simulink model "NeuromuscularModelwImpedance"  (R2014b)
settings: Solver=ode15s  StartTime=0.0  StopTime=20  MaxStep=.01  RelTol=1e-4  AbsTol=1e-6
values from neighbouring files (symbols this model uses):
  ankleAngleThr = 2*pi/180    (= 0.0349065850399)    [ControlParams.m]    (also in assignGains.m = Gains(48); saveInitialGuess.m = Gains(40))
  bKneeSwing1 = 0.02    [ControlParams.m]    (also in assignGains.m = Gains(36); saveInitialGuess.m = Gains(28))
  bKneeSwing2 = 0.03    [ControlParams.m]    (also in assignGains.m = Gains(37); saveInitialGuess.m = Gains(29))
  k1AnkleStance1 = 5*180/pi    (= 286.478897565)    [ControlParams.m]    (also in assignGains.m = Gains(38); saveInitialGuess.m = Gains(30))
  k1AnkleStance2 = 5*180/pi    (= 286.478897565)    [ControlParams.m]    (also in assignGains.m = Gains(39); saveInitialGuess.m = Gains(31))
  k1AnkleSwing1 = .5*180/pi    (= 28.6478897565)    [ControlParams.m]    (also in assignGains.m = Gains(40); saveInitialGuess.m = Gains(32))
  k1AnkleSwing2 = 0.75*180/pi    (= 42.9718346348)    [ControlParams.m]    (also in assignGains.m = Gains(41); saveInitialGuess.m = Gains(33))
  k1KneeStance1 = 3.7*180/pi    (= 211.994384198)    [ControlParams.m]    (also in assignGains.m = Gains(42); saveInitialGuess.m = Gains(34))
  k1KneeStance2 = 2.53*180/pi    (= 144.958322168)    [ControlParams.m]    (also in assignGains.m = Gains(43); saveInitialGuess.m = Gains(35))
  k1KneeSwing1 = 0.05*180/pi    (= 2.86478897565)    [ControlParams.m]    (also in assignGains.m = Gains(44); saveInitialGuess.m = Gains(36))
  k1KneeSwing2 = 2.3*180/pi    (= 131.78029288)    [ControlParams.m]    (also in assignGains.m = Gains(45); saveInitialGuess.m = Gains(37))
  k2AnkleStance1 = .5*(180/pi)^3    (= 94045.4744072)    [ControlParams.m]    (also in assignGains.m = Gains(46); saveInitialGuess.m = Gains(38))
  k2KneeStance2 = 7e-4*(180/pi)^3    (= 131.66366417)    [ControlParams.m]    (also in assignGains.m = Gains(47); saveInitialGuess.m = Gains(39))
  LceOffsetTA = 1-0.5*w    [ControlParams.m]
  legLengthClr = .9    (= 0.9)    [ControlParams.m]    (also in assignGains.m = Gains(56); saveInitialGuess.m = Gains(48))
  LongDelay = 0.020    (= 0.02)    [ControlParams.m]
  MidDelay = 0.010    (= 0.01)    [ControlParams.m]
  phiAnkleStance1 = 5*pi/180    (= 0.0872664625997)    [ControlParams.m]    (also in assignGains.m = Gains(49); saveInitialGuess.m = Gains(41))
  phiAnkleStance12 = 2*pi/180    (= 0.0349065850399)    [ControlParams.m]    (also in assignGains.m = Gains(50); saveInitialGuess.m = Gains(42))
  phiAnkleStance2 = 10*pi/180    (= 0.174532925199)    [ControlParams.m]    (also in assignGains.m = Gains(51); saveInitialGuess.m = Gains(43))
  phiHATref = 6*pi/180    (= 0.10471975512)    [ControlParams.m]
  phiKneeStance1 = 8*pi/180    (= 0.13962634016)    [ControlParams.m]    (also in assignGains.m = Gains(52); saveInitialGuess.m = Gains(44))
  phiKneeStance2 = 16*pi/180    (= 0.279252680319)    [ControlParams.m]    (also in assignGains.m = Gains(53); saveInitialGuess.m = Gains(45))
  phiKneeSwing1 = 65*pi/180    (= 1.1344640138)    [ControlParams.m]    (also in assignGains.m = Gains(54); saveInitialGuess.m = Gains(46))
  phiKneeSwing2 = 40*pi/180    (= 0.698131700798)    [ControlParams.m]    (also in assignGains.m = Gains(55); saveInitialGuess.m = Gains(47))
  PreStimGG = 0.05    [ControlParams.m]
  PreStimGLU = 0.01    [ControlParams.m]
  PreStimHAM = 0.01    [ControlParams.m]
  ShortDelay = 0.005    [ControlParams.m]
  simbiconGainD = 5*pi/180    (= 0.0872664625997)    [ControlParams.m]    (also in assignGains.m = Gains(57); saveInitialGuess.m = Gains(49))
  simbiconGainV = 5*pi/180    (= 0.0872664625997)    [ControlParams.m]    (also in assignGains.m = Gains(58); saveInitialGuess.m = Gains(50))
  simbiconLegAngle0 = 85*pi/180    (= 1.4835298642)    [ControlParams.m]    (also in assignGains.m = Gains(59); saveInitialGuess.m = Gains(51))
undefined symbols (not defined in the file or in its folder): DeltaThRef, footCenterToCGDist, footInertia, footMass, g, loptGAS, loptHAMCut, loptTA, lslackGAS, lslackHAMCut, phimaxGASa, phimaxGASk, phirefGASa, phirefGASk, phirefHAMh, rGASa, rGASk, rHAMh, rhoGASa, rhoGASk, rhoHAMh, X, Y, Z
undefined symbols (not defined in the file): RGainGLU, RGainHAM, RhipDGain, RhipPGain, RKglu, RlegAngleFilter, RPosGainGG, RSpeedGainGG
libraries: NeuroMuscularLibrary x67, nesl_utility x16, sm_lib x14, simulink x5, dspswit3 x5, simulink_extras x2
(part 2 of 2)

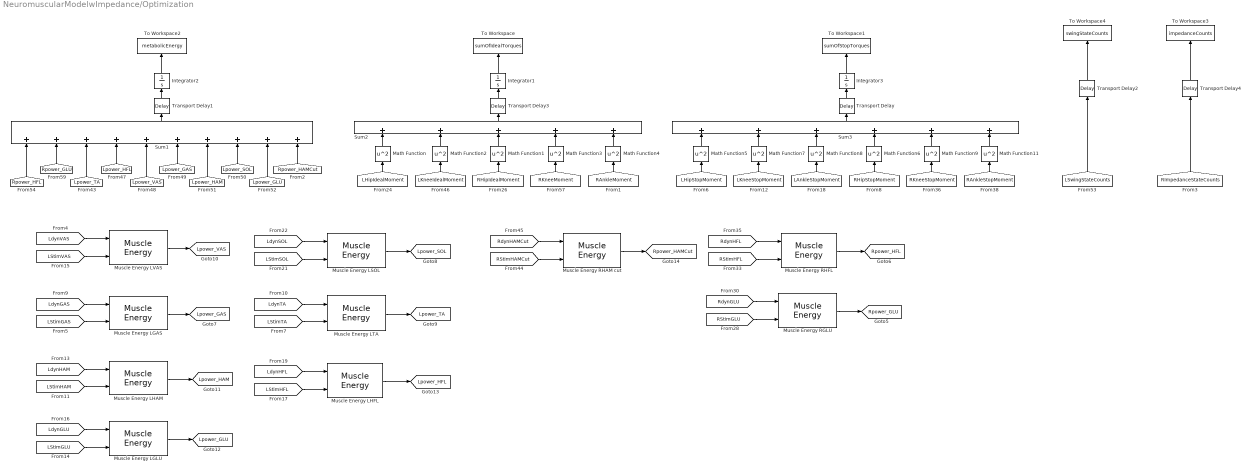
== system NeuromuscularModelwImpedance/Optimization ==
  Integrator1 : Integrator
  Integrator2 : Integrator
  Integrator3 : Integrator
  Math Function{,1..9,11} (11 alike) : Math  Operator=square  SaturateOnIntegerOverflow=on
  Muscle Energy LGAS : NeuroMuscularLibrary/Muscle Energy  lopt=loptGAS  FT=FT_GAS  Fmax=FmaxGAS
  Muscle Energy LGLU : NeuroMuscularLibrary/Muscle Energy  lopt=loptGLU  FT=FT_GLU  Fmax=FmaxGLU
  Muscle Energy LHAM : NeuroMuscularLibrary/Muscle Energy  lopt=loptHAM  FT=FT_HAM  Fmax=FmaxHAM
  Muscle Energy LHFL : NeuroMuscularLibrary/Muscle Energy  lopt=loptHFL  FT=FT_HFL  Fmax=FmaxHFL
  Muscle Energy LSOL : NeuroMuscularLibrary/Muscle Energy  lopt=loptSOL  FT=FT_SOL  Fmax=FmaxSOL
  Muscle Energy LTA : NeuroMuscularLibrary/Muscle Energy  lopt=loptTA  FT=FT_TA  Fmax=FmaxTA
  Muscle Energy LVAS : NeuroMuscularLibrary/Muscle Energy  lopt=loptVAS  FT=FT_VAS  Fmax=FmaxVAS
  Muscle Energy RGLU : NeuroMuscularLibrary/Muscle Energy  lopt=loptGLU  FT=FT_GLU  Fmax=FmaxGLU
  Muscle Energy RHAM cut : NeuroMuscularLibrary/Muscle Energy  lopt=loptHAMCut  FT=FT_HAM  Fmax=FmaxHAMCut
  Muscle Energy RHFL : NeuroMuscularLibrary/Muscle Energy  lopt=loptHFL  FT=FT_HFL  Fmax=FmaxHFL
  Sum1 : Sum  Inputs=++++++++++
  Sum2 : Sum  Inputs=+++++
  Sum3 : Sum  Inputs=++++++
  To Workspace : ToWorkspace  VariableName=sumOfIdealTorques  SampleTime=-1
      settings: MaxDataPoints=1
  To Workspace1 : ToWorkspace  VariableName=sumOfStopTorques  SampleTime=-1
      settings: MaxDataPoints=1
  To Workspace2 : ToWorkspace  VariableName=metabolicEnergy  SampleTime=-1
      settings: MaxDataPoints=1
  To Workspace3 : ToWorkspace  VariableName=impedanceCounts  SampleTime=-1
      settings: MaxDataPoints=1
  To Workspace4 : ToWorkspace  VariableName=swingStateCounts  SampleTime=-1
      settings: MaxDataPoints=1
  Transport Delay : TransportDelay  DelayTime=3  BufferSize=57344
  Transport Delay1 : TransportDelay  DelayTime=3  BufferSize=57344
  Transport Delay2 : TransportDelay  DelayTime=3  BufferSize=24576
  Transport Delay3 : TransportDelay  DelayTime=3  BufferSize=24576
  Transport Delay4 : TransportDelay  DelayTime=3  BufferSize=24576
  tag scope: Lpower_GAS=global, Lpower_GLU=global, Lpower_HAM=global, Lpower_HFL=global, Lpower_SOL=global, Lpower_TA=global, Lpower_VAS=global, Rpower_GLU=global, Rpower_HAMCut=global, Rpower_HFL=global
  wires:
  [RdynGLU] -> Muscle Energy RGLU/1
  [RStimGLU] -> Muscle Energy RGLU/2
  [RdynHFL] -> Muscle Energy RHFL/1
  [RStimHFL] -> Muscle Energy RHFL/2
  Muscle Energy RGLU/1 -> [Rpower_GLU]
  Muscle Energy RHFL/1 -> [Rpower_HFL]
  [LdynSOL] -> Muscle Energy LSOL/1
  [LStimSOL] -> Muscle Energy LSOL/2
  [LStimVAS] -> Muscle Energy LVAS/2
  [LStimGAS] -> Muscle Energy LGAS/2
  Muscle Energy LVAS/1 -> [Lpower_VAS]
  Muscle Energy LGAS/1 -> [Lpower_GAS]
  Muscle Energy LSOL/1 -> [Lpower_SOL]
  Muscle Energy LTA/1 -> [Lpower_TA]
  [LdynTA] -> Muscle Energy LTA/1
  [LStimTA] -> Muscle Energy LTA/2
  [LdynHAM] -> Muscle Energy LHAM/1
  [LStimHAM] -> Muscle Energy LHAM/2
  [LdynGLU] -> Muscle Energy LGLU/1
  [LStimGLU] -> Muscle Energy LGLU/2
  [LdynHFL] -> Muscle Energy LHFL/1
  [LStimHFL] -> Muscle Energy LHFL/2
  Muscle Energy LHAM/1 -> [Lpower_HAM]
  Muscle Energy LGLU/1 -> [Lpower_GLU]
  Muscle Energy LHFL/1 -> [Lpower_HFL]
  [LdynGAS] -> Muscle Energy LGAS/1
  [LdynVAS] -> Muscle Energy LVAS/1
  [RdynHAMCut] -> Muscle Energy RHAM cut/1
  [RStimHAMCut] -> Muscle Energy RHAM cut/2
  Muscle Energy RHAM cut/1 -> [Rpower_HAMCut]
  Integrator2/1 -> To Workspace2/1
  [Rpower_HFL] -> Sum1/1
  [Rpower_GLU] -> Sum1/2
  [Lpower_TA] -> Sum1/3
  [Lpower_HFL] -> Sum1/4
  [Lpower_VAS] -> Sum1/5
  [Lpower_GAS] -> Sum1/6
  [Lpower_HAM] -> Sum1/7
  [Lpower_SOL] -> Sum1/8
  [Lpower_GLU] -> Sum1/9
  Integrator1/1 -> To Workspace/1
  Math Function/1 -> Sum2/1
  [LHipIdealMoment] -> Math Function/1
  Math Function2/1 -> Sum2/2
  [LKneeIdealMoment] -> Math Function2/1
  [RHipIdealMoment] -> Math Function1/1
  Math Function1/1 -> Sum2/3
  [RKneeMoment] -> Math Function3/1
  Math Function3/1 -> Sum2/4
  [RAnkleMoment] -> Math Function4/1
  Math Function4/1 -> Sum2/5
  [Rpower_HAMCut] -> Sum1/10
  Integrator3/1 -> To Workspace1/1
  Math Function5/1 -> Sum3/1
  [LHipStopMoment] -> Math Function5/1
  Math Function7/1 -> Sum3/2
  [LKneeStopMoment] -> Math Function7/1
  [RHipStopMoment] -> Math Function6/1
  Math Function8/1 -> Sum3/3
  [LAnkleStopMoment] -> Math Function8/1
  Math Function6/1 -> Sum3/4
  Sum3/1 -> Transport Delay/1
  Transport Delay/1 -> Integrator3/1
  Sum1/1 -> Transport Delay1/1
  Transport Delay1/1 -> Integrator2/1
  Transport Delay3/1 -> Integrator1/1
  Sum2/1 -> Transport Delay3/1
  [LSwingStateCounts] -> Transport Delay2/1
  Transport Delay2/1 -> To Workspace4/1
  [RImpedanceStateCounts] -> Transport Delay4/1
  Transport Delay4/1 -> To Workspace3/1
  [RKneeStopMoment] -> Math Function9/1
  Math Function9/1 -> Sum3/5
  [RAnkleStopMoment] -> Math Function11/1
  Math Function11/1 -> Sum3/6

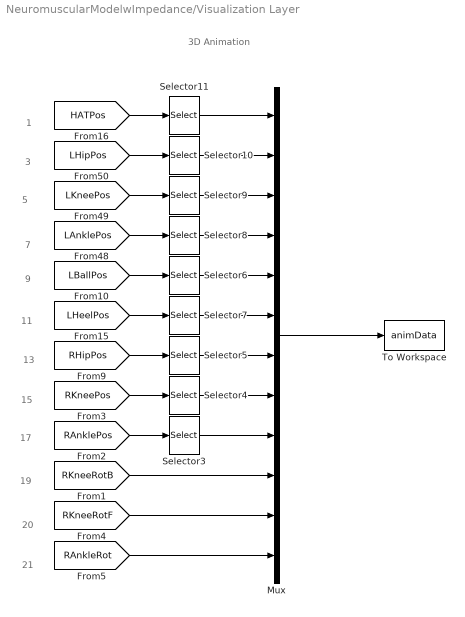
== system NeuromuscularModelwImpedance/Visualization Layer ==
  note: 20
  note: 19
  note: 17
  note: 15
  note: 13
  note: 11
  note: 9
  note: 7
  note: 5
  note: 3
  note: 1
  note: 3D Animation
  note: 21
  Mux : Mux  Inputs=12
  Selector{3..11} (9 alike) : Selector  InputPortWidth=3  Indices=[1 3]
  To Workspace : ToWorkspace  VariableName=animData  SaveFormat=Structure With Time  SampleTime=1/30
  wires:
  [RAnklePos] -> Selector3/1
  [RKneePos] -> Selector4/1
  [RHipPos] -> Selector5/1
  [HATPos] -> Selector11/1
  [LHeelPos] -> Selector7/1
  [LBallPos] -> Selector6/1
  [LAnklePos] -> Selector8/1
  [LKneePos] -> Selector9/1
  [LHipPos] -> Selector10/1
  Selector11/1 -> Mux/1
  Selector3/1 -> Mux/9
  Selector4/1 -> Mux/8
  Selector5/1 -> Mux/7
  Selector7/1 -> Mux/6
  Selector6/1 -> Mux/5
  Selector8/1 -> Mux/4
  Selector9/1 -> Mux/3
  Selector10/1 -> Mux/2
  [RKneeRotB] -> Mux/10
  [RKneeRotF] -> Mux/11
  [RAnkleRot] -> Mux/12
  Mux/1 -> To Workspace/1

== system NeuromuscularModelwImpedance/Body Mechanics Layer/HAT Speed Sensor ==
  PS-Simulink Converter1 : nesl_utility/PS-Simulink Converter  PhysicalDomain=network_engine_domain  SubClassName=ps_output  LeftPortType=input  RightPortType=output  PseudoPeriodic=off  Frequencies=[]  Unit=m/s  AffineConversion=off
  Position Sensor : sm_lib/Frames and Transforms/Transform Sensor  MeasurementFrame=World  SenseAngle=off  SenseAxis=off  SenseAngle1=off  SenseAngle2=off  SenseAngle3=off  SenseQ=off  SenseR=off  SenseOmegaX=off  SenseOmegaY=off  SenseOmegaZ=off  SenseOmega1=off  SenseOmega2=off  SenseOmega3=off  SenseQDot=off  SenseRDot=off  SenseAlphaX=off  SenseAlphaY=off  SenseAlphaZ=off  SenseAlpha1=off  SenseAlpha2=off  SenseAlpha3=off  SenseQDDot=off  SenseRDDot=off  SenseX=off  SenseY=off  SenseZ=off  SenseRad=off  SenseAzim=off  SenseDist=off  SenseInc=off  SenseXDot=on  SenseYDot=off  SenseZDot=off  SenseRadDot=off  SenseAzimDot=off  SenseDistDot=off  SenseIncDot=off  SenseXDDot=off  SenseYDDot=off  SenseZDDot=off  SenseRadDDot=off  SenseAzimDDot=off  SenseDistDDot=off  SenseIncDDot=off  BlockFunction=simmechanics.library.frames_transforms.transform_sensor
  World Frame : sm_lib/Frames and Transforms/World Frame  BlockFunction=simmechanics.library.frames_transforms.world_frame
  Frame : PMIOPort  Port=1  Side=Left
  Speed : Outport
  wires:
  PS-Simulink Converter1/1 -> Speed/1
  connections:
  Position Sensor/RConn2 -- PS-Simulink Converter1/LConn1
  Position Sensor/RConn1 -- Frame/RConn1
  Position Sensor/LConn1 -- World Frame/RConn1

== system NeuromuscularModelwImpedance/Body Mechanics Layer/Hip Pos//Speed Sensor ==
  Mux : Mux  Inputs=2
  PS-Simulink Converter : nesl_utility/PS-Simulink Converter  PhysicalDomain=network_engine_domain  SubClassName=ps_output  LeftPortType=input  RightPortType=output  PseudoPeriodic=off  Frequencies=[]  Unit=m  AffineConversion=off
  PS-Simulink Converter1 : nesl_utility/PS-Simulink Converter  PhysicalDomain=network_engine_domain  SubClassName=ps_output  LeftPortType=input  RightPortType=output  PseudoPeriodic=off  Frequencies=[]  Unit=m/s  AffineConversion=off
  Position Sensor : sm_lib/Frames and Transforms/Transform Sensor  MeasurementFrame=World  SenseAngle=off  SenseAxis=off  SenseAngle1=off  SenseAngle2=off  SenseAngle3=off  SenseQ=off  SenseR=off  SenseOmegaX=off  SenseOmegaY=off  SenseOmegaZ=off  SenseOmega1=off  SenseOmega2=off  SenseOmega3=off  SenseQDot=off  SenseRDot=off  SenseAlphaX=off  SenseAlphaY=off  SenseAlphaZ=off  SenseAlpha1=off  SenseAlpha2=off  SenseAlpha3=off  SenseQDDot=off  SenseRDDot=off  SenseX=on  SenseY=off  SenseZ=off  SenseRad=off  SenseAzim=off  SenseDist=off  SenseInc=off  SenseXDot=on  SenseYDot=off  SenseZDot=off  SenseRadDot=off  SenseAzimDot=off  SenseDistDot=off  SenseIncDot=off  SenseXDDot=off  SenseYDDot=off  SenseZDDot=off  SenseRadDDot=off  SenseAzimDDot=off  SenseDistDDot=off  SenseIncDDot=off  BlockFunction=simmechanics.library.frames_transforms.transform_sensor
  World Frame : sm_lib/Frames and Transforms/World Frame  BlockFunction=simmechanics.library.frames_transforms.world_frame
  Frame : PMIOPort  Port=1  Side=Left
  PosSpeed : Outport
  wires:
  PS-Simulink Converter1/1 -> Mux/2
  PS-Simulink Converter/1 -> Mux/1
  Mux/1 -> PosSpeed/1
  connections:
  PS-Simulink Converter1/LConn1 -- Position Sensor/RConn3
  PS-Simulink Converter/LConn1 -- Position Sensor/RConn2
  Position Sensor/RConn1 -- Frame/RConn1
  Position Sensor/LConn1 -- World Frame/RConn1

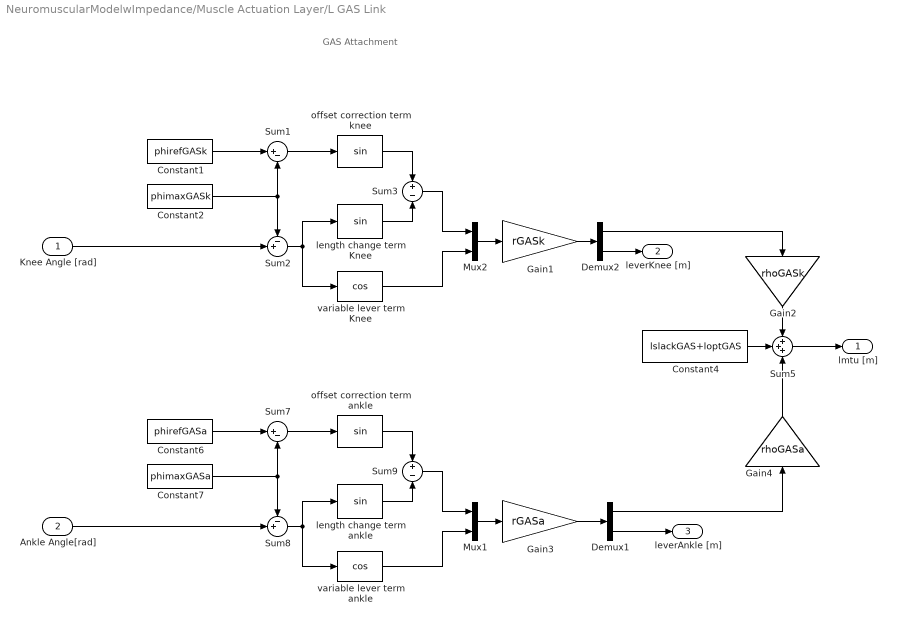
== system NeuromuscularModelwImpedance/Muscle Actuation Layer/L GAS Link ==
  note: GAS Attachment
  Knee Angle [rad] : Inport
  Ankle Angle[rad] : Inport  Port=2
  Constant1 : Constant  Value=phirefGASk
  Constant2 : Constant  Value=phimaxGASk
  Constant4 : Constant  Value=lslackGAS+loptGAS
  Constant6 : Constant  Value=phirefGASa
  Constant7 : Constant  Value=phimaxGASa
  Demux1 : Demux  Outputs=2
  Demux2 : Demux  Outputs=2
  Gain1 : Gain  Gain=rGASk
  Gain2 : Gain  Gain=rhoGASk
  Gain3 : Gain  Gain=rGASa
  Gain4 : Gain  Gain=rhoGASa
  Mux1 : Mux  Inputs=2
  Mux2 : Mux  Inputs=2
  Sum1 : Sum  Inputs=|+-
  Sum2 : Sum  Inputs=-+|
  Sum3 : Sum  Inputs=+-
  Sum5 : Sum  Inputs=+++
  Sum7 : Sum  Inputs=|+-
  Sum8 : Sum  Inputs=-+|
  Sum9 : Sum  Inputs=+-
  length change term Knee : Trigonometry
  length change term ankle : Trigonometry
  offset correction term ankle : Trigonometry
  offset correction term knee : Trigonometry
  variable lever term Knee : Trigonometry  Operator=cos
  variable lever term ankle : Trigonometry  Operator=cos
  lmtu [m] : Outport
  leverKnee [m] : Outport  Port=2
  leverAnkle [m] : Outport  Port=3
  wires:
  Gain2/1 -> Sum5/1
  Demux2/1 -> Gain2/1
  Demux2/2 -> leverKnee [m]/1
  Gain1/1 -> Demux2/1
  Mux2/1 -> Gain1/1
  Sum3/1 -> Mux2/1
  offset correction term knee/1 -> Sum3/1
  length change term Knee/1 -> Sum3/2
  Constant1/1 -> Sum1/1
  Sum1/1 -> offset correction term knee/1
  Constant2/1 -> Sum1/2, Sum2/1
  Sum2/1 -> length change term Knee/1, variable lever term Knee/1
  variable lever term Knee/1 -> Mux2/2
  Knee Angle [rad]/1 -> Sum2/2
  Gain4/1 -> Sum5/3
  Demux1/1 -> Gain4/1
  Gain3/1 -> Demux1/1
  Mux1/1 -> Gain3/1
  Constant4/1 -> Sum5/2
  Sum9/1 -> Mux1/1
  offset correction term ankle/1 -> Sum9/1
  length change term ankle/1 -> Sum9/2
  Constant6/1 -> Sum7/1
  Sum7/1 -> offset correction term ankle/1
  Constant7/1 -> Sum7/2, Sum8/1
  Sum8/1 -> length change term ankle/1, variable lever term ankle/1
  Demux1/2 -> leverAnkle [m]/1
  variable lever term ankle/1 -> Mux1/2
  Sum5/1 -> lmtu [m]/1
  Ankle Angle[rad]/1 -> Sum8/2

== system NeuromuscularModelwImpedance/Muscle Actuation Layer/R HAM Link Cut ==
  note: HAM Attachment
  hip angle : Inport
  Constant3 : Constant  Value=rHAMh
  Constant4 : Constant  Value=lslackHAMCut+loptHAMCut
  Constant5 : Constant  Value=phirefHAMh
  Gain2 : Gain  Gain=rhoHAMh
  Product : Product  RndMeth=Zero
  Sum4 : Sum  Inputs=|+-
  Sum5 : Sum  Inputs=-+
  lmtu : Outport
  hip lever [m] : Outport  Port=2
  wires:
  Constant5/1 -> Sum4/2
  Sum4/1 -> Product/1
  Constant3/1 -> hip lever [m]/1, Product/2
  Product/1 -> Gain2/1
  Sum5/1 -> lmtu/1
  Constant4/1 -> Sum5/2
  Gain2/1 -> Sum5/1
  hip angle/1 -> Sum4/1

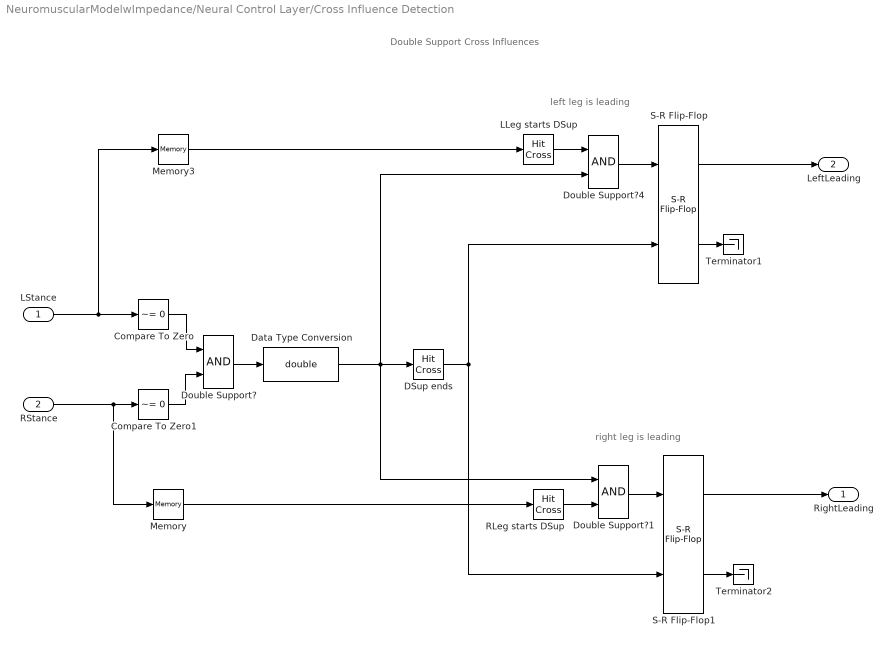
== system NeuromuscularModelwImpedance/Neural Control Layer/Cross Influence Detection ==
  note: Double Support Cross Influences
  note: left leg is leading
  note: right leg is leading
  LStance : Inport
  RStance : Inport  Port=2
  Compare To Zero : simulink/Logic and Bit Operations/Compare To Zero  relop=~=  OutDataTypeStr=boolean
  Compare To Zero1 : simulink/Logic and Bit Operations/Compare To Zero  relop=~=  OutDataTypeStr=boolean
  DSup ends : HitCross  HitCrossingOffset=0.5  HitCrossingDirection=falling  ZeroCross=off
  Data Type Conversion : DataTypeConversion  OutDataTypeStr=double
  Double Support? : Logic  AllPortsSameDT=off
  Double Support?1 : Logic  AllPortsSameDT=off
  Double Support?4 : Logic  AllPortsSameDT=off
  LLeg starts DSup : HitCross  HitCrossingOffset=0.5  HitCrossingDirection=rising  ZeroCross=off
  Memory : Memory
  Memory3 : Memory
  RLeg starts DSup : HitCross  HitCrossingOffset=0.5  HitCrossingDirection=rising  ZeroCross=off
  S-R Flip-Flop : simulink_extras/Flip Flops/S-R Flip-Flop  initial_condition=0
  S-R Flip-Flop1 : simulink_extras/Flip Flops/S-R Flip-Flop  initial_condition=0
  Terminator1 : Terminator
  Terminator2 : Terminator
  RightLeading : Outport
  LeftLeading : Outport  Port=2
  wires:
  Data Type Conversion/1 -> DSup ends/1, Double Support?4/2, Double Support?1/1
  Double Support?/1 -> Data Type Conversion/1
  Compare To Zero1/1 -> Double Support?/2
  Compare To Zero/1 -> Double Support?/1
  DSup ends/1 -> S-R Flip-Flop1/2, S-R Flip-Flop/2
  Double Support?4/1 -> S-R Flip-Flop/1
  LLeg starts DSup/1 -> Double Support?4/1
  Memory3/1 -> LLeg starts DSup/1
  Double Support?1/1 -> S-R Flip-Flop1/1
  RLeg starts DSup/1 -> Double Support?1/2
  Memory/1 -> RLeg starts DSup/1
  S-R Flip-Flop1/1 -> RightLeading/1
  RStance/1 -> Memory/1, Compare To Zero1/1
  LStance/1 -> Compare To Zero/1, Memory3/1
  S-R Flip-Flop1/2 -> Terminator2/1
  S-R Flip-Flop/1 -> LeftLeading/1
  S-R Flip-Flop/2 -> Terminator1/1

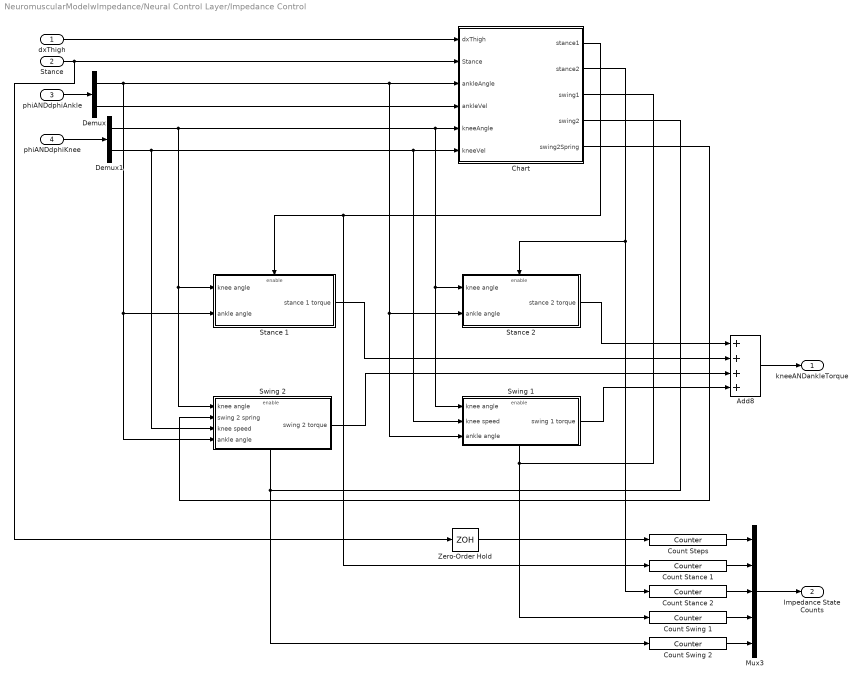
== system NeuromuscularModelwImpedance/Neural Control Layer/Impedance Control ==
  dxThigh : Inport
  Stance : Inport  Port=2
  phiANDdphiAnkle : Inport  Port=3
  phiANDdphiKnee : Inport  Port=4
  Add8 : Sum  Inputs=++++
  Chart : Stateflow chart  TreatAsAtomicUnit=on
  Count Stance 1 : dspswit3/Counter  Direction=Up  CountEvent=Rising edge  CounterSize=16 bits  MaxCount=255  InitialCount=0  Output=Count  HitValue=32  ResetInput=off  SamplesPerFrame=1  Ts=1  CntDtype=double  HitDtype=Logical
  Count Stance 2 : dspswit3/Counter  Direction=Up  CountEvent=Rising edge  CounterSize=16 bits  MaxCount=255  InitialCount=0  Output=Count  HitValue=32  ResetInput=off  SamplesPerFrame=1  Ts=1  CntDtype=double  HitDtype=Logical
  Count Steps : dspswit3/Counter  Direction=Up  CountEvent=Rising edge  CounterSize=16 bits  MaxCount=255  InitialCount=0  Output=Count  HitValue=32  ResetInput=off  SamplesPerFrame=1  Ts=1  CntDtype=double  HitDtype=Logical
  Count Swing 1 : dspswit3/Counter  Direction=Up  CountEvent=Rising edge  CounterSize=16 bits  MaxCount=255  InitialCount=0  Output=Count  HitValue=32  ResetInput=off  SamplesPerFrame=1  Ts=1  CntDtype=double  HitDtype=Logical
  Count Swing 2 : dspswit3/Counter  Direction=Up  CountEvent=Rising edge  CounterSize=16 bits  MaxCount=255  InitialCount=0  Output=Count  HitValue=32  ResetInput=off  SamplesPerFrame=1  Ts=1  CntDtype=double  HitDtype=Logical
  Demux : Demux  Outputs=2
  Demux1 : Demux  Outputs=2
  Mux3 : Mux  Inputs=5
  Stance 1 : Subsystem
  Stance 2 : Subsystem
  Swing 1 : Subsystem
  Swing 2 : Subsystem
  Zero-Order Hold : ZeroOrderHold  SampleTime=.01
  kneeANDankleTorque : Outport
  Impedance State Counts : Outport  Port=2
  wires:
  phiANDdphiAnkle/1 -> Demux/1
  phiANDdphiKnee/1 -> Demux1/1
  Demux/2 -> Chart/4(ankleVel)
  Demux/1 -> Chart/3(ankleAngle), Stance 2/2(ankle angle), Swing 1/3(ankle angle), Swing 2/4(ankle angle), Stance 1/2(ankle angle)
  Add8/1 -> kneeANDankleTorque/1
  Stance 2/1(stance 2 torque) -> Add8/1
  Stance 1/1(stance 1 torque) -> Add8/2
  Swing 1/1(swing 1 torque) -> Add8/4
  Swing 2/1(swing 2 torque) -> Add8/3
  Chart/1(stance1) -> Count Stance 1/1, Stance 1/Enable
  Chart/2(stance2) -> Count Stance 2/1, Stance 2/Enable
  Chart/3(swing1) -> Count Swing 1/1, Swing 1/Enable
  Chart/4(swing2) -> Swing 2/Enable, Count Swing 2/1
  dxThigh/1 -> Chart/1(dxThigh)
  Demux1/1 -> Swing 2/1(knee angle), Stance 1/1(knee angle), Swing 1/1(knee angle), Stance 2/1(knee angle), Chart/5(kneeAngle)
  Demux1/2 -> Swing 2/3(knee speed), Swing 1/2(knee speed), Chart/6(kneeVel)
  Chart/5(swing2Spring) -> Swing 2/2(swing 2 spring)
  Stance/1 -> Zero-Order Hold/1, Chart/2(Stance)
  Count Swing 2/1 -> Mux3/5
  Count Swing 1/1 -> Mux3/4
  Count Stance 2/1 -> Mux3/3
  Count Stance 1/1 -> Mux3/2
  Mux3/1 -> Impedance State Counts/1
  Count Steps/1 -> Mux3/1
  Zero-Order Hold/1 -> Count Steps/1

== system NeuromuscularModelwImpedance/Neural Control Layer/Right Hard Stops ==
  Ideal Torques : Inport
  Muscle Torques : Inport  Port=2
  phiANDdphiHip : Inport  Port=3
  Add : Sum  Inputs=+++
  Demux1 : Demux  Outputs=2
  Hip Overextension Joint Limit : NeuroMuscularLibrary/Overextension Joint Limit  phiUpLimit=phiHipUpLimit  ext=1
  Net Torque : Outport
  Hip Stop Torque : Outport  Port=2
  wires:
  Muscle Torques/1 -> Add/2
  Demux1/1 -> Hip Overextension Joint Limit/1
  Demux1/2 -> Hip Overextension Joint Limit/2
  Hip Overextension Joint Limit/1 -> Add/3, Hip Stop Torque/1
  phiANDdphiHip/1 -> Demux1/1
  Add/1 -> Net Torque/1
  Ideal Torques/1 -> Add/1

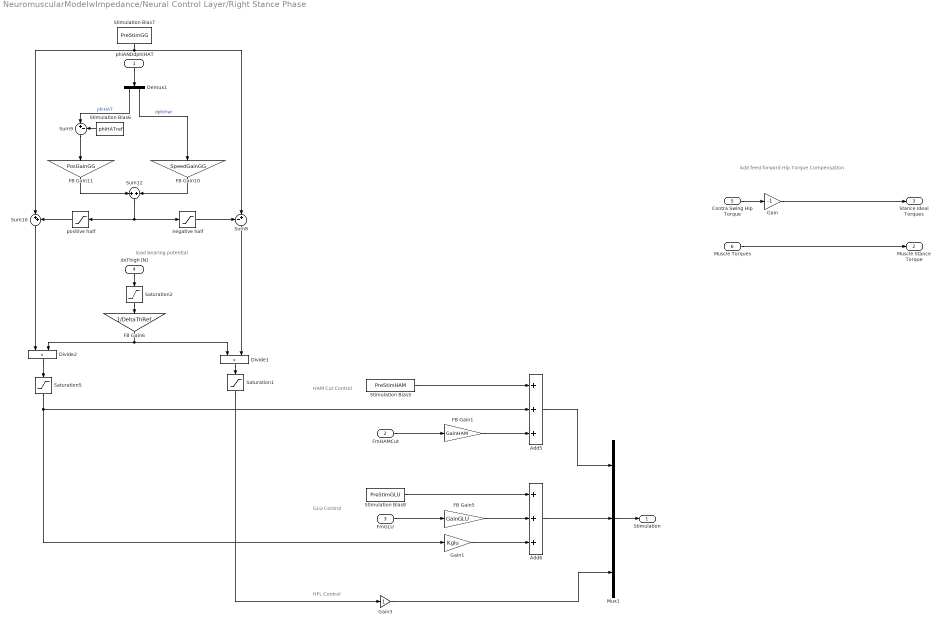
== system NeuromuscularModelwImpedance/Neural Control Layer/Right Stance Phase ==
  note: load bearing potential
  note: HFL Control
  note: GLU Control
  note: HAM Cut Control
  note: Add feed forward Hip Torque Compensation
  phiANDdphiHAT : Inport
  FmHAMCut : Inport  Port=2
  FmGLU : Inport  Port=3
  dxThigh [N] : Inport  Port=4
  Contra Swing Hip Torque : Inport  Port=5
  Muscle Torques : Inport  Port=6
  Add5 : Sum  Inputs=+++
  Add6 : Sum  Inputs=+++
  Demux1 : Demux  Outputs=2
  Divide1 : Product
  Divide2 : Product
  FB Gain1 : Gain  Gain=GainHAM  SaturateOnIntegerOverflow=on  OutDataTypeStr=Inherit: Same as input  ParamDataTypeStr=Inherit: Same as input
  FB Gain10 : Gain  Gain=SpeedGainGG  SaturateOnIntegerOverflow=on  OutDataTypeStr=Inherit: Same as input  ParamDataTypeStr=Inherit: Same as input
  FB Gain11 : Gain  Gain=PosGainGG  SaturateOnIntegerOverflow=on  OutDataTypeStr=Inherit: Same as input  ParamDataTypeStr=Inherit: Same as input
  FB Gain5 : Gain  Gain=GainGLU  SaturateOnIntegerOverflow=on  OutDataTypeStr=Inherit: Same as input  ParamDataTypeStr=Inherit: Same as input
  FB Gain6 : Gain  Gain=1/DeltaThRef  SaturateOnIntegerOverflow=on  OutDataTypeStr=Inherit: Same as input  ParamDataTypeStr=Inherit: Same as input
  Gain : Gain  Gain=-1
  Gain1 : Gain  Gain=Kglu
  Gain3 : Gain
  Mux1 : Mux  Inputs=3
  Saturation1 : Saturate  UpperLimit=1  LowerLimit=0  ZeroCross=off
  Saturation2 : Saturate  UpperLimit=inf  LowerLimit=0  ZeroCross=off
  Saturation5 : Saturate  UpperLimit=1  LowerLimit=0  ZeroCross=off
  Stimulation Bias5 : Constant  Value=PreStimHAM
  Stimulation Bias6 : Constant  Value=phiHATref
  Stimulation Bias7 : Constant  Value=PreStimGG
  Stimulation Bias8 : Constant  Value=PreStimGLU
  Sum10 : Sum  Inputs=|++  SaturateOnIntegerOverflow=on  InputSameDT=on  OutDataTypeStr=Inherit: Same as first input
  Sum12 : Sum  SaturateOnIntegerOverflow=on  InputSameDT=on  OutDataTypeStr=Inherit: Same as first input
  Sum8 : Sum  Inputs=-+|  SaturateOnIntegerOverflow=on  InputSameDT=on  OutDataTypeStr=Inherit: Same as first input
  Sum9 : Sum  Inputs=|+-  SaturateOnIntegerOverflow=on  InputSameDT=on  OutDataTypeStr=Inherit: Same as first input
  negative half : Saturate  UpperLimit=0  LowerLimit=-inf  ZeroCross=off
  positive half : Saturate  UpperLimit=inf  LowerLimit=0  ZeroCross=off
  Stimulation : Outport
  Muscle Stance Torque : Outport  Port=2
  Stance Ideal Torques : Outport  Port=3
  wires:
  Mux1/1 -> Stimulation/1
  Gain1/1 -> Add6/3
  FB Gain5/1 -> Add6/2
  Stimulation Bias8/1 -> Add6/1
  Add6/1 -> Mux1/2
  Add5/1 -> Mux1/1
  FB Gain1/1 -> Add5/3
  Stimulation Bias5/1 -> Add5/1
  FmGLU/1 -> FB Gain5/1
  FmHAMCut/1 -> FB Gain1/1
  Sum8/1 -> Divide1/2
  Sum10/1 -> Divide2/1
  Sum9/1 -> FB Gain11/1
  FB Gain6/1 -> Divide1/1, Divide2/2
  Saturation5/1 -> Add5/2, Gain1/1
  Divide2/1 -> Saturation5/1
  Divide1/1 -> Saturation1/1
  Saturation1/1 -> Gain3/1
  dxThigh [N]/1 -> Saturation2/1
  Saturation2/1 -> FB Gain6/1
  Gain3/1 -> Mux1/3
  negative half/1 -> Sum8/1
  Sum12/1 -> negative half/1, positive half/1
  positive half/1 -> Sum10/2
  Demux1/2 -> FB Gain10/1  "dphiHat"
  Demux1/1 -> Sum9/1  "phiHAT"
  phiANDdphiHAT/1 -> Demux1/1
  FB Gain10/1 -> Sum12/2
  FB Gain11/1 -> Sum12/1
  Stimulation Bias7/1 -> Sum8/2, Sum10/1
  Stimulation Bias6/1 -> Sum9/2
  Muscle Torques/1 -> Muscle Stance Torque/1
  Gain/1 -> Stance Ideal Torques/1
  Contra Swing Hip Torque/1 -> Gain/1

== system NeuromuscularModelwImpedance/Neural Control Layer/Right Swing Phase ==
  note: Stimulation
  note: Torques
  Muscle Torques : Inport
  Leg Angle : Inport  Port=2
  H Target Leg Angle : Inport  Port=3
  " 2" : Gain  Gain=0
  " 3" : Gain  Gain=hipPGain
  " 4" : Gain  Gain=hipDGain
  Add2 : Sum  Inputs=+-
  Constant6 : Constant  Value=zeros(3,1)
  Filtered Derivative : NeuroMuscularLibrary/Swing Phase/Filtered Derivative
  Sum1 : Sum  Inputs=|+-
  Wait 100 ms to enable : NeuroMuscularLibrary/Swing Phase/Wait 100 ms to enable
  Stimulation : Outport
  Torques : Outport  Port=2
  Swing Muscle Torques : Outport  Port=3
  wires:
  Constant6/1 -> Stimulation/1
  Add2/1 -> Torques/1  "Hip Torque"
  Sum1/1 -> " 3"/1
  " 3"/1 -> Add2/1
  " 4"/1 -> Add2/2
  H Target Leg Angle/1 -> Sum1/1
  Filtered Derivative/1 -> Wait 100 ms to enable/1
  Wait 100 ms to enable/1 -> " 4"/1
  Leg Angle/1 -> Sum1/2, Filtered Derivative/1
  Muscle Torques/1 -> " 2"/1
  " 2"/1 -> Swing Muscle Torques/1

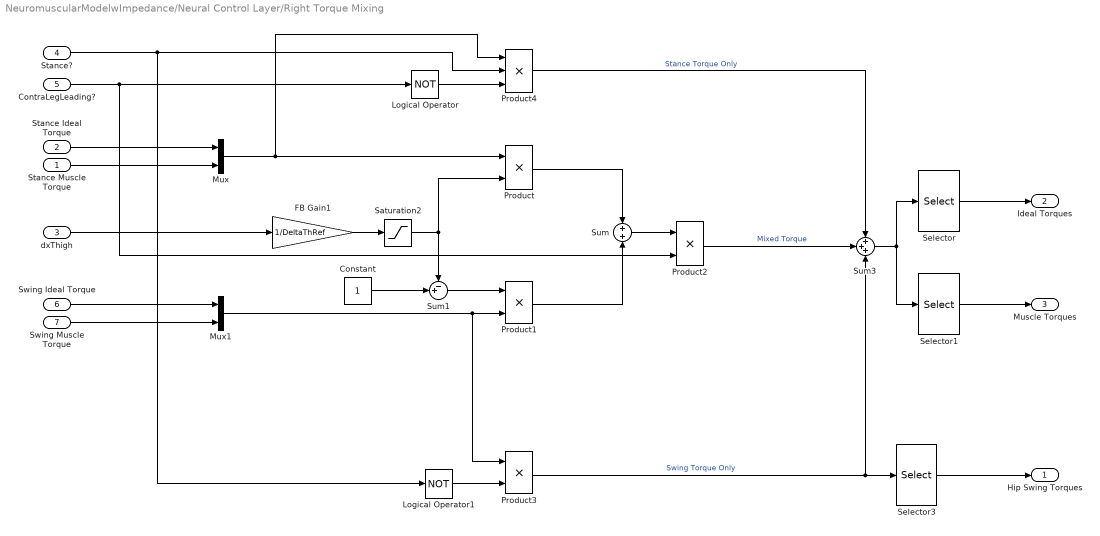
== system NeuromuscularModelwImpedance/Neural Control Layer/Right Torque Mixing ==
  Stance Muscle Torque : Inport
  Stance Ideal Torque : Inport  Port=2
  dxThigh : Inport  Port=3
  Stance? : Inport  Port=4
  ContraLegLeading? : Inport  Port=5
  Swing Ideal Torque : Inport  Port=6
  Swing Muscle Torque : Inport  Port=7
  Constant : Constant
  FB Gain1 : Gain  Gain=1/DeltaThRef  SaturateOnIntegerOverflow=on  OutDataTypeStr=Inherit: Same as input  ParamDataTypeStr=Inherit: Same as input
  Logical Operator : Logic  Operator=NOT  AllPortsSameDT=off  OutDataTypeStr=boolean
  Logical Operator1 : Logic  Operator=NOT  AllPortsSameDT=off  OutDataTypeStr=boolean
  Mux : Mux  Inputs=2
  Mux1 : Mux  Inputs=2
  Product{,1..3} (4 alike) : Product
  Product4 : Product  Inputs=3
  Saturation2 : Saturate  UpperLimit=1  LowerLimit=0  ZeroCross=off
  Selector : Selector  InputPortWidth=2  Indices=[1]
  Selector1 : Selector  InputPortWidth=2  Indices=[2]
  Selector3 : Selector  InputPortWidth=2
  Sum : Sum  Inputs=+|+
  Sum1 : Sum  Inputs=-+|
  Sum3 : Sum  Inputs=+++
  Hip Swing Torques : Outport  OutputWhenDisabled=reset
  Ideal Torques : Outport  Port=2  OutputWhenDisabled=reset
  Muscle Torques : Outport  Port=3  OutputWhenDisabled=reset
  wires:
  Selector3/1 -> Hip Swing Torques/1
  Sum3/1 -> Selector/1, Selector1/1
  Selector1/1 -> Muscle Torques/1
  Selector/1 -> Ideal Torques/1
  Swing Muscle Torque/1 -> Mux1/2
  Swing Ideal Torque/1 -> Mux1/1
  Stance Muscle Torque/1 -> Mux/2
  Stance Ideal Torque/1 -> Mux/1
  dxThigh/1 -> FB Gain1/1
  Mux/1 -> Product4/1, Product/1
  FB Gain1/1 -> Saturation2/1
  Saturation2/1 -> Product/2, Sum1/1
  Mux1/1 -> Product1/2, Product3/1
  Constant/1 -> Sum1/2
  Sum1/1 -> Product1/1
  Product1/1 -> Sum/2
  Product/1 -> Sum/1
  Logical Operator/1 -> Product4/3
  Stance?/1 -> Logical Operator1/1, Product4/2
  Sum/1 -> Product2/1
  Product2/1 -> Sum3/2  "Mixed Torque"
  Product4/1 -> Sum3/1  "Stance Torque Only"
  Logical Operator1/1 -> Product3/2
  Product3/1 -> Sum3/3, Selector3/1  "Swing Torque Only"
  ContraLegLeading?/1 -> Product2/2, Logical Operator/1

== system NeuromuscularModelwImpedance/Neural Control Layer/simbicon target leg angle ==
  LeftAnklePos : Inport
  HIPposAndSpeed : Inport  Port=2
  RightAnklePos : Inport  Port=3
  Add : Sum  Inputs=+++
  Add1 : Sum  Inputs=+++
  Constant : Constant  Value=simbiconLegAngle0
  Demux : Demux  Outputs=2
  Gain : Gain  Gain=-simbiconGainD
  Gain1 : Gain  Gain=-simbiconGainD
  Gain2 : Gain  Gain=-simbiconGainV
  Selector : Selector  InputPortWidth=3  Indices=[1]
  Selector1 : Selector  InputPortWidth=3  Indices=[1]
  Sum : Sum  Inputs=|-+
  Sum1 : Sum  Inputs=+-|
  Left Target Leg Angle : Outport
  Right Target Leg Angle : Outport  Port=2
  wires:
  Demux/2 -> Gain2/1  "Hip x speed"
  Selector1/1 -> Sum1/2
  RightAnklePos/1 -> Selector1/1
  Selector/1 -> Sum/1
  LeftAnklePos/1 -> Selector/1
  Add/1 -> Right Target Leg Angle/1
  Add1/1 -> Left Target Leg Angle/1
  Constant/1 -> Add1/1, Add/1
  Gain1/1 -> Add1/3
  Gain2/1 -> Add/3, Add1/2
  Gain/1 -> Add/2
  Sum1/1 -> Gain1/1
  Sum/1 -> Gain/1
  Demux/1 -> Sum1/1, Sum/2  "Hip x pos"
  HIPposAndSpeed/1 -> Demux/1

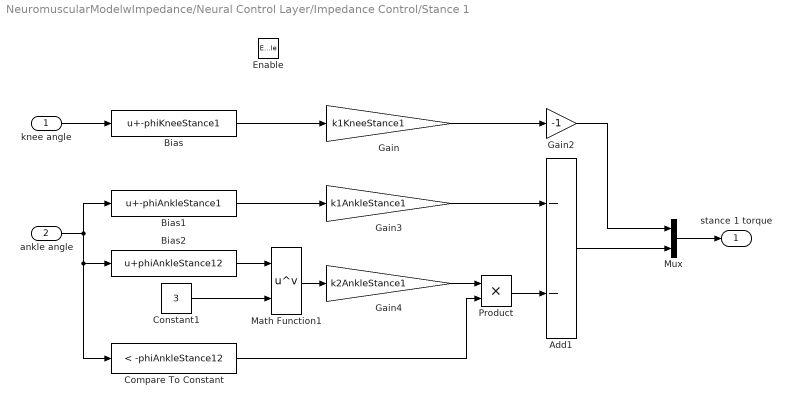
== system NeuromuscularModelwImpedance/Neural Control Layer/Impedance Control/Stance 1 ==
  knee angle : Inport
  ankle angle : Inport  Port=2
  Enable : EnablePort  StatesWhenEnabling=reset
  Add1 : Sum  Inputs=--
  Bias : Bias  Bias=-phiKneeStance1
  Bias1 : Bias  Bias=-phiAnkleStance1
  Bias2 : Bias  Bias=phiAnkleStance12
  Compare To Constant : simulink/Logic and Bit Operations/Compare To Constant  relop=<  const=-phiAnkleStance12  OutDataTypeStr=boolean  ZeroCross=off
  Constant1 : Constant  Value=3
  Gain : Gain  Gain=k1KneeStance1
  Gain2 : Gain  Gain=-1
  Gain3 : Gain  Gain=k1AnkleStance1
  Gain4 : Gain  Gain=k2AnkleStance1
  Math Function1 : Math  Operator=pow  SaturateOnIntegerOverflow=on
  Mux : Mux  Inputs=2
  Product : Product
  stance 1 torque : Outport  OutputWhenDisabled=reset  InitialOutput=[0 0]
  wires:
  Constant1/1 -> Math Function1/2
  Bias/1 -> Gain/1
  Mux/1 -> stance 1 torque/1
  Add1/1 -> Mux/2
  Gain3/1 -> Add1/1
  Bias1/1 -> Gain3/1
  Math Function1/1 -> Gain4/1
  Gain/1 -> Gain2/1
  Gain2/1 -> Mux/1
  ankle angle/1 -> Bias1/1, Compare To Constant/1, Bias2/1
  knee angle/1 -> Bias/1
  Bias2/1 -> Math Function1/1
  Gain4/1 -> Product/1
  Product/1 -> Add1/2
  Compare To Constant/1 -> Product/2

== system NeuromuscularModelwImpedance/Neural Control Layer/Impedance Control/Stance 2 ==
  knee angle : Inport
  ankle angle : Inport  Port=2
  Enable : EnablePort  StatesWhenEnabling=reset
  Add2 : Sum  Inputs=--
  Bias2 : Bias  Bias=-phiKneeStance2
  Bias3 : Bias  Bias=-phiAnkleStance2
  Constant2 : Constant  Value=3
  Gain5 : Gain  Gain=-1
  Gain6 : Gain  Gain=k1KneeStance2
  Gain7 : Gain  Gain=k2KneeStance2
  Gain9 : Gain  Gain=k1AnkleStance2
  Math Function2 : Math  Operator=pow  SaturateOnIntegerOverflow=on
  Mux1 : Mux  Inputs=2
  stance 2 torque : Outport  OutputWhenDisabled=reset  InitialOutput=[0 0]
  wires:
  Gain6/1 -> Add2/1
  Math Function2/1 -> Gain7/1
  Gain9/1 -> Gain5/1
  Bias3/1 -> Gain9/1
  Constant2/1 -> Math Function2/2
  Bias2/1 -> Math Function2/1, Gain6/1
  Gain7/1 -> Add2/2
  Add2/1 -> Mux1/1
  Mux1/1 -> stance 2 torque/1
  Gain5/1 -> Mux1/2
  ankle angle/1 -> Bias3/1
  knee angle/1 -> Bias2/1

== system NeuromuscularModelwImpedance/Neural Control Layer/Impedance Control/Swing 1 ==
  knee angle : Inport
  knee speed : Inport  Port=2
  ankle angle : Inport  Port=3
  Enable : EnablePort  StatesWhenEnabling=reset
  Add3 : Sum  Inputs=--
  Bias6 : Bias  Bias=-phiKneeSwing1
  Gain20 : Gain  Gain=k1KneeSwing1
  Gain22 : Gain  Gain=bKneeSwing1
  Gain23 : Gain  Gain=k1AnkleSwing1
  Gain8 : Gain  Gain=-1
  Mux3 : Mux  Inputs=2
  swing 1 torque : Outport  OutputWhenDisabled=reset  InitialOutput=[0 0]
  wires:
  Bias6/1 -> Gain20/1
  Gain20/1 -> Add3/1
  Gain22/1 -> Add3/2
  Gain23/1 -> Gain8/1
  ankle angle/1 -> Gain23/1
  Add3/1 -> Mux3/1
  Gain8/1 -> Mux3/2
  knee angle/1 -> Bias6/1
  knee speed/1 -> Gain22/1
  Mux3/1 -> swing 1 torque/1

== system NeuromuscularModelwImpedance/Neural Control Layer/Impedance Control/Swing 2 ==
  knee angle : Inport
  swing 2 spring : Inport  Port=2
  knee speed : Inport  Port=3
  ankle angle : Inport  Port=4
  Enable : EnablePort  StatesWhenEnabling=reset
  Add4 : Sum  Inputs=--
  Bias4 : Bias  Bias=-phiKneeSwing2
  Gain1 : Gain  Gain=-1
  Gain12 : Gain  Gain=k1KneeSwing2
  Gain16 : Gain  Gain=bKneeSwing2
  Gain17 : Gain  Gain=k1AnkleSwing2
  Mux2 : Mux  Inputs=2
  Product : Product
  swing 2 torque : Outport  OutputWhenDisabled=reset  InitialOutput=[0 0]
  wires:
  Bias4/1 -> Gain12/1
  ankle angle/1 -> Gain17/1
  Gain17/1 -> Gain1/1
  Gain16/1 -> Add4/2
  Gain1/1 -> Mux2/2
  Add4/1 -> Mux2/1
  Mux2/1 -> swing 2 torque/1
  knee speed/1 -> Gain16/1
  knee angle/1 -> Bias4/1
  Product/1 -> Add4/1
  Gain12/1 -> Product/1
  swing 2 spring/1 -> Product/2

== stateflow chart NeuromuscularModelwImpedance/Neural Control Layer/Impedance Control/Chart ==
  state Stance1
    entry: stance1 = 1;
    exit: stance1 = 0;
  state Stance2
    entry: stance2 = 1;
    exit: stance2 = 0;
  state Swing2
    entry: swing2 = 1;
    exit: swing2 = 0;
    state Swing2SpringOFF
      entry: swing2Spring = 0;
    state Swing2SpringON
      entry: swing2Spring = 1;
    Swing2SpringOFF -> Swing2SpringON : [kneeAngle < phiKneeSwing2]
    (default) -> Swing2SpringOFF
  state Swing1
    entry: swing1 = 1;
    exit: swing1 = 0;
  Stance1 -> Stance2 : [(ankleAngle < -ankleAngleThr) && (ankleVel > 0)]
  Swing1 -> Stance1 [order 2] : [Stance && dxThigh > DeltaThRef/2]
  Swing2 -> Stance1 : [Stance && dxThigh > DeltaThRef/2]
  Stance2 -> Swing1 : [~Stance]
  Swing1 -> Swing2 [order 1] : [kneeVel < 0]
  (default) -> Swing2
  data: dxThigh input; Stance input; DeltaThRef parameter; ankleAngle input; ankleVel input; kneeAngle input; kneeVel input; stance1 output; stance2 output; swing1 output; swing2 output; ankleAngleThr parameter; swing2Spring output double; phiKneeSwing2 parameter
